simulink model "gm_CustArch"  (R2020a)
settings: Solver=FixedStepDiscrete  StartTime=0.0  StopTime=7e4  RelTol=1e-3
libraries: simulink x85, hdlsllib x52, hdlmdlgenlib x2
(part 3 of 3)

== system gm_CustArch/cust_architecture/process_and_retrieve/80-120Hz IIR/controlss_temp/Filter/delay_process_section12_tap1 ==
  in0 : Inport  OutDataTypeStr=fixdt(1, 16, 15)  SampleTime=1
  Trigger_emulated : EnablePort  OutDataTypeStr=boolean
  delay_process_section12_tap1 : Delay  DelayLength=double(1)
  out0 : Outport  OutDataTypeStr=fixdt(1, 16, 15)  InitialOutput=0
  wires:
  delay_process_section12_tap1/1 -> out0/1
  in0/1 -> delay_process_section12_tap1/1

== system gm_CustArch/cust_architecture/process_and_retrieve/80-120Hz IIR/controlss_temp/Filter/delay_process_section13_tap0 ==
  in0 : Inport  OutDataTypeStr=fixdt(1, 16, 15)  SampleTime=1
  Trigger_emulated : EnablePort  OutDataTypeStr=boolean
  delay_process_section13_tap0 : Delay  DelayLength=double(1)
  out0 : Outport  OutDataTypeStr=fixdt(1, 16, 15)  InitialOutput=0
  wires:
  delay_process_section13_tap0/1 -> out0/1
  in0/1 -> delay_process_section13_tap0/1

== system gm_CustArch/cust_architecture/process_and_retrieve/80-120Hz IIR/controlss_temp/Filter/delay_process_section13_tap1 ==
  in0 : Inport  OutDataTypeStr=fixdt(1, 16, 15)  SampleTime=1
  Trigger_emulated : EnablePort  OutDataTypeStr=boolean
  delay_process_section13_tap1 : Delay  DelayLength=double(1)
  out0 : Outport  OutDataTypeStr=fixdt(1, 16, 15)  InitialOutput=0
  wires:
  delay_process_section13_tap1/1 -> out0/1
  in0/1 -> delay_process_section13_tap1/1

== system gm_CustArch/cust_architecture/process_and_retrieve/80-120Hz IIR/controlss_temp/Filter/delay_process_section14_tap0 ==
  in0 : Inport  OutDataTypeStr=fixdt(1, 16, 15)  SampleTime=1
  Trigger_emulated : EnablePort  OutDataTypeStr=boolean
  delay_process_section14_tap0 : Delay  DelayLength=double(1)
  out0 : Outport  OutDataTypeStr=fixdt(1, 16, 15)  InitialOutput=0
  wires:
  delay_process_section14_tap0/1 -> out0/1
  in0/1 -> delay_process_section14_tap0/1

== system gm_CustArch/cust_architecture/process_and_retrieve/80-120Hz IIR/controlss_temp/Filter/delay_process_section14_tap1 ==
  in0 : Inport  OutDataTypeStr=fixdt(1, 16, 15)  SampleTime=1
  Trigger_emulated : EnablePort  OutDataTypeStr=boolean
  delay_process_section14_tap1 : Delay  DelayLength=double(1)
  out0 : Outport  OutDataTypeStr=fixdt(1, 16, 15)  InitialOutput=0
  wires:
  delay_process_section14_tap1/1 -> out0/1
  in0/1 -> delay_process_section14_tap1/1

== system gm_CustArch/cust_architecture/process_and_retrieve/80-120Hz IIR/controlss_temp/Filter/delay_process_section15_tap0 ==
  in0 : Inport  OutDataTypeStr=fixdt(1, 16, 15)  SampleTime=1
  Trigger_emulated : EnablePort  OutDataTypeStr=boolean
  delay_process_section15_tap0 : Delay  DelayLength=double(1)
  out0 : Outport  OutDataTypeStr=fixdt(1, 16, 15)  InitialOutput=0
  wires:
  delay_process_section15_tap0/1 -> out0/1
  in0/1 -> delay_process_section15_tap0/1

== system gm_CustArch/cust_architecture/process_and_retrieve/80-120Hz IIR/controlss_temp/Filter/delay_process_section15_tap1 ==
  in0 : Inport  OutDataTypeStr=fixdt(1, 16, 15)  SampleTime=1
  Trigger_emulated : EnablePort  OutDataTypeStr=boolean
  delay_process_section15_tap1 : Delay  DelayLength=double(1)
  out0 : Outport  OutDataTypeStr=fixdt(1, 16, 15)  InitialOutput=0
  wires:
  delay_process_section15_tap1/1 -> out0/1
  in0/1 -> delay_process_section15_tap1/1

== system gm_CustArch/cust_architecture/process_and_retrieve/80-120Hz IIR/controlss_temp/Filter/delay_process_section16_tap0 ==
  in0 : Inport  OutDataTypeStr=fixdt(1, 16, 15)  SampleTime=1
  Trigger_emulated : EnablePort  OutDataTypeStr=boolean
  delay_process_section16_tap0 : Delay  DelayLength=double(1)
  out0 : Outport  OutDataTypeStr=fixdt(1, 16, 15)  InitialOutput=0
  wires:
  delay_process_section16_tap0/1 -> out0/1
  in0/1 -> delay_process_section16_tap0/1

== system gm_CustArch/cust_architecture/process_and_retrieve/80-120Hz IIR/controlss_temp/Filter/delay_process_section16_tap1 ==
  in0 : Inport  OutDataTypeStr=fixdt(1, 16, 15)  SampleTime=1
  Trigger_emulated : EnablePort  OutDataTypeStr=boolean
  delay_process_section16_tap1 : Delay  DelayLength=double(1)
  out0 : Outport  OutDataTypeStr=fixdt(1, 16, 15)  InitialOutput=0
  wires:
  delay_process_section16_tap1/1 -> out0/1
  in0/1 -> delay_process_section16_tap1/1

== system gm_CustArch/cust_architecture/process_and_retrieve/80-120Hz IIR/controlss_temp/Filter/delay_process_section17_tap0 ==
  in0 : Inport  OutDataTypeStr=fixdt(1, 16, 15)  SampleTime=1
  Trigger_emulated : EnablePort  OutDataTypeStr=boolean
  delay_process_section17_tap0 : Delay  DelayLength=double(1)
  out0 : Outport  OutDataTypeStr=fixdt(1, 16, 15)  InitialOutput=0
  wires:
  delay_process_section17_tap0/1 -> out0/1
  in0/1 -> delay_process_section17_tap0/1

== system gm_CustArch/cust_architecture/process_and_retrieve/80-120Hz IIR/controlss_temp/Filter/delay_process_section17_tap1 ==
  in0 : Inport  OutDataTypeStr=fixdt(1, 16, 15)  SampleTime=1
  Trigger_emulated : EnablePort  OutDataTypeStr=boolean
  delay_process_section17_tap1 : Delay  DelayLength=double(1)
  out0 : Outport  OutDataTypeStr=fixdt(1, 16, 15)  InitialOutput=0
  wires:
  delay_process_section17_tap1/1 -> out0/1
  in0/1 -> delay_process_section17_tap1/1

== system gm_CustArch/cust_architecture/process_and_retrieve/80-120Hz IIR/controlss_temp/Filter/delay_process_section18_tap0 ==
  in0 : Inport  OutDataTypeStr=fixdt(1, 16, 15)  SampleTime=1
  Trigger_emulated : EnablePort  OutDataTypeStr=boolean
  delay_process_section18_tap0 : Delay  DelayLength=double(1)
  out0 : Outport  OutDataTypeStr=fixdt(1, 16, 15)  InitialOutput=0
  wires:
  delay_process_section18_tap0/1 -> out0/1
  in0/1 -> delay_process_section18_tap0/1

== system gm_CustArch/cust_architecture/process_and_retrieve/80-120Hz IIR/controlss_temp/Filter/delay_process_section18_tap1 ==
  in0 : Inport  OutDataTypeStr=fixdt(1, 16, 15)  SampleTime=1
  Trigger_emulated : EnablePort  OutDataTypeStr=boolean
  delay_process_section18_tap1 : Delay  DelayLength=double(1)
  out0 : Outport  OutDataTypeStr=fixdt(1, 16, 15)  InitialOutput=0
  wires:
  delay_process_section18_tap1/1 -> out0/1
  in0/1 -> delay_process_section18_tap1/1

== system gm_CustArch/cust_architecture/process_and_retrieve/80-120Hz IIR/controlss_temp/Filter/delay_process_section1_tap0 ==
  in0 : Inport  OutDataTypeStr=fixdt(1, 16, 15)  SampleTime=1
  Trigger_emulated : EnablePort  OutDataTypeStr=boolean
  delay_process_section1_tap0 : Delay  DelayLength=double(1)
  out0 : Outport  OutDataTypeStr=fixdt(1, 16, 15)  InitialOutput=0
  wires:
  delay_process_section1_tap0/1 -> out0/1
  in0/1 -> delay_process_section1_tap0/1

== system gm_CustArch/cust_architecture/process_and_retrieve/80-120Hz IIR/controlss_temp/Filter/delay_process_section1_tap1 ==
  in0 : Inport  OutDataTypeStr=fixdt(1, 16, 15)  SampleTime=1
  Trigger_emulated : EnablePort  OutDataTypeStr=boolean
  delay_process_section1_tap1 : Delay  DelayLength=double(1)
  out0 : Outport  OutDataTypeStr=fixdt(1, 16, 15)  InitialOutput=0
  wires:
  delay_process_section1_tap1/1 -> out0/1
  in0/1 -> delay_process_section1_tap1/1

== system gm_CustArch/cust_architecture/process_and_retrieve/80-120Hz IIR/controlss_temp/Filter/delay_process_section2_tap0 ==
  in0 : Inport  OutDataTypeStr=fixdt(1, 16, 15)  SampleTime=1
  Trigger_emulated : EnablePort  OutDataTypeStr=boolean
  delay_process_section2_tap0 : Delay  DelayLength=double(1)
  out0 : Outport  OutDataTypeStr=fixdt(1, 16, 15)  InitialOutput=0
  wires:
  delay_process_section2_tap0/1 -> out0/1
  in0/1 -> delay_process_section2_tap0/1

== system gm_CustArch/cust_architecture/process_and_retrieve/80-120Hz IIR/controlss_temp/Filter/delay_process_section2_tap1 ==
  in0 : Inport  OutDataTypeStr=fixdt(1, 16, 15)  SampleTime=1
  Trigger_emulated : EnablePort  OutDataTypeStr=boolean
  delay_process_section2_tap1 : Delay  DelayLength=double(1)
  out0 : Outport  OutDataTypeStr=fixdt(1, 16, 15)  InitialOutput=0
  wires:
  delay_process_section2_tap1/1 -> out0/1
  in0/1 -> delay_process_section2_tap1/1

== system gm_CustArch/cust_architecture/process_and_retrieve/80-120Hz IIR/controlss_temp/Filter/delay_process_section3_tap0 ==
  in0 : Inport  OutDataTypeStr=fixdt(1, 16, 15)  SampleTime=1
  Trigger_emulated : EnablePort  OutDataTypeStr=boolean
  delay_process_section3_tap0 : Delay  DelayLength=double(1)
  out0 : Outport  OutDataTypeStr=fixdt(1, 16, 15)  InitialOutput=0
  wires:
  delay_process_section3_tap0/1 -> out0/1
  in0/1 -> delay_process_section3_tap0/1

== system gm_CustArch/cust_architecture/process_and_retrieve/80-120Hz IIR/controlss_temp/Filter/delay_process_section3_tap1 ==
  in0 : Inport  OutDataTypeStr=fixdt(1, 16, 15)  SampleTime=1
  Trigger_emulated : EnablePort  OutDataTypeStr=boolean
  delay_process_section3_tap1 : Delay  DelayLength=double(1)
  out0 : Outport  OutDataTypeStr=fixdt(1, 16, 15)  InitialOutput=0
  wires:
  delay_process_section3_tap1/1 -> out0/1
  in0/1 -> delay_process_section3_tap1/1

== system gm_CustArch/cust_architecture/process_and_retrieve/80-120Hz IIR/controlss_temp/Filter/delay_process_section4_tap0 ==
  in0 : Inport  OutDataTypeStr=fixdt(1, 16, 15)  SampleTime=1
  Trigger_emulated : EnablePort  OutDataTypeStr=boolean
  delay_process_section4_tap0 : Delay  DelayLength=double(1)
  out0 : Outport  OutDataTypeStr=fixdt(1, 16, 15)  InitialOutput=0
  wires:
  delay_process_section4_tap0/1 -> out0/1
  in0/1 -> delay_process_section4_tap0/1

== system gm_CustArch/cust_architecture/process_and_retrieve/80-120Hz IIR/controlss_temp/Filter/delay_process_section4_tap1 ==
  in0 : Inport  OutDataTypeStr=fixdt(1, 16, 15)  SampleTime=1
  Trigger_emulated : EnablePort  OutDataTypeStr=boolean
  delay_process_section4_tap1 : Delay  DelayLength=double(1)
  out0 : Outport  OutDataTypeStr=fixdt(1, 16, 15)  InitialOutput=0
  wires:
  delay_process_section4_tap1/1 -> out0/1
  in0/1 -> delay_process_section4_tap1/1

== system gm_CustArch/cust_architecture/process_and_retrieve/80-120Hz IIR/controlss_temp/Filter/delay_process_section5_tap0 ==
  in0 : Inport  OutDataTypeStr=fixdt(1, 16, 15)  SampleTime=1
  Trigger_emulated : EnablePort  OutDataTypeStr=boolean
  delay_process_section5_tap0 : Delay  DelayLength=double(1)
  out0 : Outport  OutDataTypeStr=fixdt(1, 16, 15)  InitialOutput=0
  wires:
  delay_process_section5_tap0/1 -> out0/1
  in0/1 -> delay_process_section5_tap0/1

== system gm_CustArch/cust_architecture/process_and_retrieve/80-120Hz IIR/controlss_temp/Filter/delay_process_section5_tap1 ==
  in0 : Inport  OutDataTypeStr=fixdt(1, 16, 15)  SampleTime=1
  Trigger_emulated : EnablePort  OutDataTypeStr=boolean
  delay_process_section5_tap1 : Delay  DelayLength=double(1)
  out0 : Outport  OutDataTypeStr=fixdt(1, 16, 15)  InitialOutput=0
  wires:
  delay_process_section5_tap1/1 -> out0/1
  in0/1 -> delay_process_section5_tap1/1

== system gm_CustArch/cust_architecture/process_and_retrieve/80-120Hz IIR/controlss_temp/Filter/delay_process_section6_tap0 ==
  in0 : Inport  OutDataTypeStr=fixdt(1, 16, 15)  SampleTime=1
  Trigger_emulated : EnablePort  OutDataTypeStr=boolean
  delay_process_section6_tap0 : Delay  DelayLength=double(1)
  out0 : Outport  OutDataTypeStr=fixdt(1, 16, 15)  InitialOutput=0
  wires:
  delay_process_section6_tap0/1 -> out0/1
  in0/1 -> delay_process_section6_tap0/1

== system gm_CustArch/cust_architecture/process_and_retrieve/80-120Hz IIR/controlss_temp/Filter/delay_process_section6_tap1 ==
  in0 : Inport  OutDataTypeStr=fixdt(1, 16, 15)  SampleTime=1
  Trigger_emulated : EnablePort  OutDataTypeStr=boolean
  delay_process_section6_tap1 : Delay  DelayLength=double(1)
  out0 : Outport  OutDataTypeStr=fixdt(1, 16, 15)  InitialOutput=0
  wires:
  delay_process_section6_tap1/1 -> out0/1
  in0/1 -> delay_process_section6_tap1/1

== system gm_CustArch/cust_architecture/process_and_retrieve/80-120Hz IIR/controlss_temp/Filter/delay_process_section7_tap0 ==
  in0 : Inport  OutDataTypeStr=fixdt(1, 16, 15)  SampleTime=1
  Trigger_emulated : EnablePort  OutDataTypeStr=boolean
  delay_process_section7_tap0 : Delay  DelayLength=double(1)
  out0 : Outport  OutDataTypeStr=fixdt(1, 16, 15)  InitialOutput=0
  wires:
  delay_process_section7_tap0/1 -> out0/1
  in0/1 -> delay_process_section7_tap0/1

== system gm_CustArch/cust_architecture/process_and_retrieve/80-120Hz IIR/controlss_temp/Filter/delay_process_section7_tap1 ==
  in0 : Inport  OutDataTypeStr=fixdt(1, 16, 15)  SampleTime=1
  Trigger_emulated : EnablePort  OutDataTypeStr=boolean
  delay_process_section7_tap1 : Delay  DelayLength=double(1)
  out0 : Outport  OutDataTypeStr=fixdt(1, 16, 15)  InitialOutput=0
  wires:
  delay_process_section7_tap1/1 -> out0/1
  in0/1 -> delay_process_section7_tap1/1

== system gm_CustArch/cust_architecture/process_and_retrieve/80-120Hz IIR/controlss_temp/Filter/delay_process_section8_tap0 ==
  in0 : Inport  OutDataTypeStr=fixdt(1, 16, 15)  SampleTime=1
  Trigger_emulated : EnablePort  OutDataTypeStr=boolean
  delay_process_section8_tap0 : Delay  DelayLength=double(1)
  out0 : Outport  OutDataTypeStr=fixdt(1, 16, 15)  InitialOutput=0
  wires:
  delay_process_section8_tap0/1 -> out0/1
  in0/1 -> delay_process_section8_tap0/1

== system gm_CustArch/cust_architecture/process_and_retrieve/80-120Hz IIR/controlss_temp/Filter/delay_process_section8_tap1 ==
  in0 : Inport  OutDataTypeStr=fixdt(1, 16, 15)  SampleTime=1
  Trigger_emulated : EnablePort  OutDataTypeStr=boolean
  delay_process_section8_tap1 : Delay  DelayLength=double(1)
  out0 : Outport  OutDataTypeStr=fixdt(1, 16, 15)  InitialOutput=0
  wires:
  delay_process_section8_tap1/1 -> out0/1
  in0/1 -> delay_process_section8_tap1/1

== system gm_CustArch/cust_architecture/process_and_retrieve/80-120Hz IIR/controlss_temp/Filter/delay_process_section9_tap0 ==
  in0 : Inport  OutDataTypeStr=fixdt(1, 16, 15)  SampleTime=1
  Trigger_emulated : EnablePort  OutDataTypeStr=boolean
  delay_process_section9_tap0 : Delay  DelayLength=double(1)
  out0 : Outport  OutDataTypeStr=fixdt(1, 16, 15)  InitialOutput=0
  wires:
  delay_process_section9_tap0/1 -> out0/1
  in0/1 -> delay_process_section9_tap0/1

== system gm_CustArch/cust_architecture/process_and_retrieve/80-120Hz IIR/controlss_temp/Filter/delay_process_section9_tap1 ==
  in0 : Inport  OutDataTypeStr=fixdt(1, 16, 15)  SampleTime=1
  Trigger_emulated : EnablePort  OutDataTypeStr=boolean
  delay_process_section9_tap1 : Delay  DelayLength=double(1)
  out0 : Outport  OutDataTypeStr=fixdt(1, 16, 15)  InitialOutput=0
  wires:
  delay_process_section9_tap1/1 -> out0/1
  in0/1 -> delay_process_section9_tap1/1

== stateflow chart gm_CustArch/cust_architecture/output_interpret/OutputStateMachine/OutputStateMachine ==
  settings: sampleTime=1/1e6  stateMachineType=MOORE_MACHINE  initializeOutput=1
  state idle_state
    OutputState=16
  state state_magic_number_0
    OutputState=0
  state state_magic_number_01
    OutputState=1
  state state_magic_number_02
    OutputState=2
  state state_magic_number_03
    OutputState=3
  state state_timestamp_0
    OutputState=4
  state state_timestamp_01
    OutputState=5
  state state_DC_sample
    OutputState=6
    count_chs=count_chs+1
  state state_chan_sample
    OutputState=7
  state state_stim_on_off
    OutputState=8
    count_chs=0
    count_stim_on_off=count_stim_on_off+1
  state state_stim_pol
    OutputState=9
    count_stim_on_off=0
    count_stim_pol=count_stim_pol+1
  state state_amp_settle
    OutputState=10
    count_stim_pol=0
    count_amp_settle=count_amp_settle+1
  state state_charge_recov
    OutputState=11
    count_amp_settle=0
    count_state_charge=count_state_charge+1
  state state_DAC
    OutputState=12
    count_state_charge=0
    count_1=count_1+1
  state state_ADC
    OutputState=13
    count_1=0
    count_2=count_2+1
  state state_TTL_in
    count_2=0
    OutputState=14
  state state_TTL_out
    OutputState=15
  (default) -> idle_state
  state_TTL_out -> idle_state
  idle_state -> state_magic_number_0 : [input_state==8]
  state_magic_number_0 -> state_magic_number_01
  state_magic_number_01 -> state_magic_number_02
  state_magic_number_02 -> state_magic_number_03
  state_magic_number_03 -> state_timestamp_0
  state_timestamp_0 -> state_timestamp_01
  state_timestamp_01 -> state_DC_sample
  state_chan_sample -> state_DC_sample [order 1] : [count_chs<160]
  state_DC_sample -> state_chan_sample
  state_chan_sample -> state_stim_on_off [order 2] : [count_chs==160]
  state_stim_on_off -> state_stim_pol : [count_stim_on_off==8]
  state_stim_pol -> state_amp_settle : [count_stim_pol==8]
  state_amp_settle -> state_charge_recov : [count_amp_settle==8]
  state_charge_recov -> state_DAC : [count_state_charge==8]
  state_DAC -> state_DAC [order 2]
  state_DAC -> state_ADC [order 1] : [count_1==8]
  state_ADC -> state_ADC [order 2]
  state_ADC -> state_TTL_in [order 1] : [count_2==8]
  state_TTL_in -> state_TTL_out
  data: OutputState output uint8 =uint8(0); count_1 local uint8 =uint8(0); count_2 local uint8 =uint8(0); input_state input uint8; count_stim_pol local uint8 =uint8(0); count_stim_on_off local uint8 =uint8(0); count_amp_settle local uint8 =uint8(0); count_state_charge local uint8 =uint8(0); count_chs local uint8 =uint8(0)

== stateflow chart gm_CustArch/cust_architecture/input_interpret_store_retrieve/InputStateMachine/InputStateMachine ==
  settings: sampleTime=1/1e6  stateMachineType=MOORE_MACHINE  initializeOutput=1
  state state_magic_number_0
    InputState=0
  state state_magic_number_01
    InputState=1
  state state_magic_number_02
    InputState=2
  state state_magic_number_03
    InputState=3
  state state_timestamp_0
    InputState=4
  state state_timestamp_01
    InputState=5
  state state_DC_sample
    InputState=6
  state state_chan_sample
    InputState=7
  state state_stim_on_off
    InputState=8
  state state_stim_pol
    InputState=9
  state state_amp_settle
    InputState=10
  state state_charge_recov
    InputState=11
  state state_DAC1
    InputState=12
    count_1=count_1
  state state_DAC
    InputState=12
    count_1=count_1+1
  note: Bad state machine?
      | Probably I should use converter counter but it works
      | so let's keep like this for now
  state state_ADC
    InputState=13
    count_1=0
    count_2=count_2+1
  state state_ADC1
    InputState=13
    count_1=0
    count_2=count_2
  state state_TTL_in
    count_2=0
    InputState=14
  state state_TTL_out
    InputState=15
  (default) -> state_magic_number_0
  state_TTL_out -> state_magic_number_0
  state_magic_number_03 -> state_magic_number_0 [order 2]
  state_timestamp_0 -> state_magic_number_0 [order 2]
  state_magic_number_02 -> state_magic_number_0 [order 2]
  state_magic_number_01 -> state_magic_number_0 [order 2]
  state_magic_number_0 -> state_magic_number_01 : [FIFO_data_in==12043 &  FIFO_write_to==1]
  state_magic_number_01 -> state_magic_number_02 [order 1] : [FIFO_data_in==18801 &  FIFO_write_to==1]
  state_magic_number_02 -> state_magic_number_03 [order 1] : [FIFO_data_in==11402 &  FIFO_write_to==1]
  state_magic_number_03 -> state_timestamp_0 [order 1] : [FIFO_data_in==36180 &  FIFO_write_to==1]
  state_timestamp_0 -> state_timestamp_01 [order 1] : [FIFO_write_to==1]
  state_timestamp_01 -> state_DC_sample : [FIFO_write_to==1]
  state_chan_sample -> state_DC_sample [order 1] : [channel_0_19<20 & FIFO_write_to==1]
  state_DC_sample -> state_stim_on_off [order 2] : [channel_0_19==20 ]
  state_DC_sample -> state_chan_sample [order 1] : [FIFO_write_to==1 & channel_0_19<20]
  state_chan_sample -> state_stim_on_off [order 2] : [channel_0_19==20 & inc_source_device_MSB==1 & FIFO_write_to==1]
  state_stim_on_off -> state_stim_pol : [inc_source_device_MSB==1]
  state_stim_pol -> state_amp_settle : [inc_source_device_MSB==1]
  state_amp_settle -> state_charge_recov : [ inc_source_device_MSB==1]
  state_charge_recov -> state_DAC : [inc_source_device_MSB==1]
  state_DAC -> state_DAC1 [order 3] : [FIFO_write_to==0]
  state_DAC -> state_DAC [order 2] : [FIFO_write_to==1]
  state_DAC1 -> state_DAC : [FIFO_write_to==1]
  state_DAC -> state_ADC [order 1] : [count_1==8]
  state_ADC -> state_ADC1 [order 3] : [FIFO_write_to==0]
  state_ADC -> state_ADC [order 2] : [FIFO_write_to==1]
  state_ADC1 -> state_ADC : [FIFO_write_to==1]
  state_ADC -> state_TTL_in [order 1] : [count_2==8]
  state_TTL_in -> state_TTL_out : [FIFO_write_to==1]
  data: FIFO_data_in input; FIFO_write_to input; InputState output uint8; channel_0_19 input; count_1 local uint8 [0..8] =uint8(0); count_2 local uint8 [0..8] =uint8(0); inc_source_device_MSB input
